simulink model "Modelnm"  (Simulink 8.5)
settings: Solver=ode45  StartTime=0.0  StopTime=0.1  RelTol=1e-3
values from neighbouring files (symbols this model uses):
  u1nm = U1nm(j,i+1)+100    [EDMC.m]    (also in EDMC_with_Constraint.m; Vri.m)
  u2nm = U2nm(j,i+1)+100    [EDMC.m]    (also in EDMC_with_Constraint.m; Vri.m)
  x01nm = x1nm(end)    [EDMC.m]    (also in EDMC_with_Constraint.m; Vri.m)
  x02nm = x2nm(end)    [EDMC.m]    (also in EDMC_with_Constraint.m; Vri.m)
settings Model: Creator=Default  LastModifiedBy=Default
settings DataIOCC: SignalLoggingSaveFormat=Dataset
settings OptimizationCC: ExpressionDepthLimit=128
settings DebuggingCC: UnderspecifiedInitializationDetection=Simplified  MergeDetectMultiDrivingBlocksExec=error  FcnCallInpInsideContextMsg=EnableAllAsError  StateNameClashWarn=none
settings GRTTargetCC: CombineOutputUpdateFcns=on  GRTInterface=off

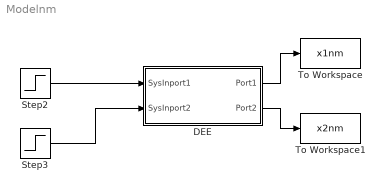
== system Modelnm ==
  DEE : Subsystem  mask(Differential Equation Editor (DEE)){}
      settings: OpenFcn=diffeqed
      mask Display: disp('Differential Equation\n Editor')
  Step2 : Step  Time=0  After=u1nm  SampleTime=0
  Step3 : Step  Time=0  After=u2nm  SampleTime=0
  To Workspace : ToWorkspace  VariableName=x1nm  SampleTime=-1
  To Workspace1 : ToWorkspace  VariableName=x2nm  SampleTime=-1
  wires:
  Step2/1 -> DEE/1(SysInport1)
  DEE/1(Port1) -> To Workspace/1
  DEE/2(Port2) -> To Workspace1/1
  Step3/1 -> DEE/2(SysInport2)

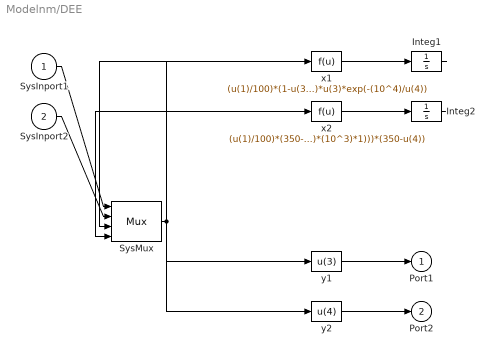
== system Modelnm/DEE ==
  SysInport1 : Inport
  SysInport2 : Inport  Port=2
  Integ1 : Integrator  InitialCondition=x01nm
  Integ2 : Integrator  InitialCondition=x02nm
  SysMux : Mux
  x1 : Fcn  Expr=(u(1)/100)*(1-u(3))-(7.2*10^10)*u(3)*exp(-(10^4)/u(4))
  x2 : Fcn  Expr=(u(1)/100)*(350-u(4))-((-(2*10^5)/(10^3))*(7.2*10^10)*u(3)*exp(-(10^4)/u(4)))+(((10^3)*1)/((10^3)*100))*(u(2))*(1-exp(-(7*10^5)/(u(2)*(10^3)*1)))*(350-u(4))
  y1 : Fcn  Expr=u(3)
  y2 : Fcn  Expr=u(4)
  Port1 : Outport
  Port2 : Outport  Port=2
  wires:
  SysInport1/1 -> SysMux/1
  SysInport2/1 -> SysMux/2
  SysMux/1 -> x1/1, x2/1, y1/1, y2/1
  x1/1 -> Integ1/1
  Integ1/1 -> SysMux/3
  x2/1 -> Integ2/1
  Integ2/1 -> SysMux/4
  y1/1 -> Port1/1
  y2/1 -> Port2/1
